simulink model "math_model_with_pid_2015a_the_newest"  (R2015a)
settings: Solver=ode3  SolverMode=SingleTasking  StartTime=0.0  StopTime=30  FixedStep=0.01  RelTol=1e-3
values from neighbouring files (symbols this model uses):
  f_c = 1.0942    [clean_pendulum_setup.m]
  f_p = 0.10436    [clean_pendulum_setup.m]
  g = 9.8101    [Wahadlo_setup.m]    (also in clean_pendulum_setup.m = 9.81)
  I = 1/12 * m_pw * l_c ^ 2      + 1/4 * m_pw * r_c ^ 2      + m_pw * l_c0 ^ 2      + 1/12 * m_ps * l_p ^ 2      + 1/4 * m_pw * r_p ^ 2      + m_ps * l_p0 ^ 2    (= 0.00542605689)    [clean_pendulum_setup.m]
  L = 0.2899    [clean_pendulum_setup.m]
  M = 0.503 + 0.045    (= 0.548)    [clean_pendulum_setup.m]
  m = m_c + m_p    (= 63.548)    [Wahadlo_setup.m]    (also in clean_pendulum_setup.m = 0.063)
  theta0 = pi/10    (= 0.314159265359)    [clean_pendulum_setup.m]
  theta_fin = 0    [clean_pendulum_setup.m]
  theta_max = pi    (= 3.14159265359)    [clean_pendulum_setup.m]
  x0 = -0.3    [clean_pendulum_setup.m]
  x_fin = 0    [clean_pendulum_setup.m]
  x_max = 0.75    [clean_pendulum_setup.m]
libraries: simulink x2
settings Model: CovMetricSettings=dwe  CovHtmlReporting=off  covSaveCumulativeToWorkspaceVar=off  CovSaveSingleToWorkspaceVar=off  CovExternalEMLEnable=on  Creator=spika  LastModifiedBy=Student
settings DataIOCC: LimitDataPoints=off  SaveFormat=Dataset  ReturnWorkspaceOutputs=on
settings DebuggingCC: SFUnexpectedBacktrackingDiag=error  SFNoUnconditionalDefaultTransitionDiag=error
settings HardwareCC: ProdBitPerPointer=64  ProdLargestAtomicFloat=Float  ProdIntDivRoundTo=Zero  ProdEndianess=LittleEndian  ProdHWDeviceType=Specified
settings ModelReferenceCC: PropagateSignalLabelsOutOfModel=on
settings SFSimCC: SimUseLocalCustomCode=on
settings RTWCC: RTWUseLocalCustomCode=on
settings GRTTargetCC: TargetLangStandard=C99 (ISO)

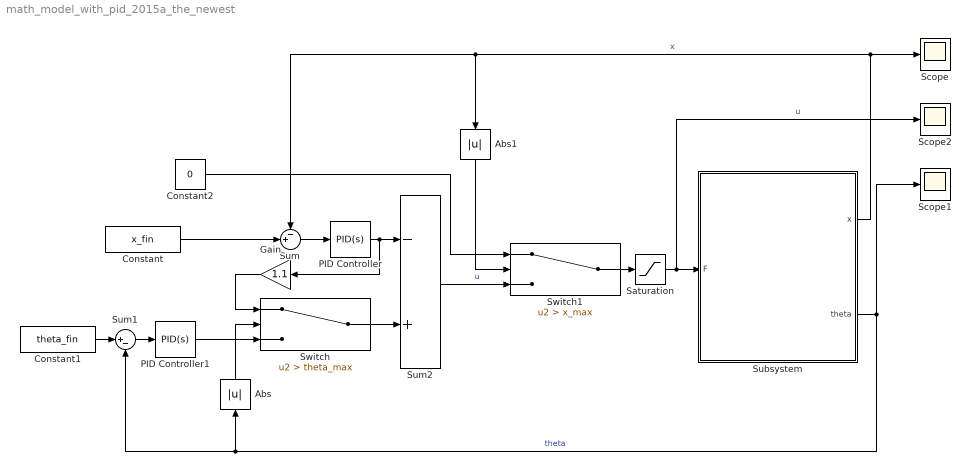
== system math_model_with_pid_2015a_the_newest ==
  Abs : Abs
  Abs1 : Abs
  Constant : Constant  Value=x_fin
  Constant1 : Constant  Value=theta_fin
  Constant2 : Constant  Value=0
  Gain : Gain  Gain=1.1
  PID Controller : simulink/Continuous/PID Controller  Controller=PID  TimeDomain=Continuous-time  SampleTime=-1  IntegratorMethod=Forward Euler  FilterMethod=Forward Euler  Form=Parallel  UseFilter=on  ControllerParametersSource=internal  P=0.9314  I=0  D=3.29  N=1.41571080218282  InitialConditionSource=internal  InitialConditionForIntegrator=0  InitialConditionForFilter=0  ExternalReset=none  LimitOutput=off  UpperSaturationLimit=inf  LowerSaturationLimit=-inf  LinearizeAsGain=on  AntiWindupMode=none  Kb=1  TrackingMode=off  Kt=1  PParamMin=[]  PParamMax=[]  IParamMin=[]  IParamMax=[]  DParamMin=[]  DParamMax=[]  NParamMin=[]  NParamMax=[]  KbParamMin=[]  KbParamMax=[]  KtParamMin=[]  KtParamMax=[]  POutMin=[]  POutMax=[]  IOutMin=[]  IOutMax=[]  DOutMin=[]  DOutMax=[]  NOutMin=[]  NOutMax=[]  KbOutMin=[]  KbOutMax=[]  KtOutMin=[]  KtOutMax=[]  IntegratorOutMin=[]  IntegratorOutMax=[]  FilterOutMin=[]  FilterOutMax=[]  SumOutMin=[]  SumOutMax=[]  SumI1OutMin=[]  SumI1OutMax=[]  SumI2OutMin=[]  SumI2OutMax=[]  SumI3OutMin=[]  SumI3OutMax=[]  SumDOutMin=[]  SumDOutMax=[]  SaturationOutMin=[]  SaturationOutMax=[]  IntegratorContinuousStateAttributes=''  IntegratorStateMustResolveToSignalObject=off  IntegratorRTWStateStorageClass=Auto  FilterContinuousStateAttributes=''  FilterStateMustResolveToSignalObject=off  FilterRTWStateStorageClass=Auto  DifferentiatorICPrevScaledInput=0  DifferentiatorOutMin=[]  DifferentiatorOutMax=[]
  PID Controller1 : simulink/Continuous/PID Controller  Controller=PID  TimeDomain=Continuous-time  SampleTime=-1  IntegratorMethod=Forward Euler  FilterMethod=Forward Euler  Form=Parallel  UseFilter=on  ControllerParametersSource=internal  P=-35  I=0  D=10  N=0.2  InitialConditionSource=internal  InitialConditionForIntegrator=0  InitialConditionForFilter=0  ExternalReset=none  LimitOutput=off  UpperSaturationLimit=inf  LowerSaturationLimit=-inf  LinearizeAsGain=on  AntiWindupMode=none  Kb=1  TrackingMode=off  Kt=1  PParamMin=[]  PParamMax=[]  IParamMin=[]  IParamMax=[]  DParamMin=[]  DParamMax=[]  NParamMin=[]  NParamMax=[]  KbParamMin=[]  KbParamMax=[]  KtParamMin=[]  KtParamMax=[]  POutMin=[]  POutMax=[]  IOutMin=[]  IOutMax=[]  DOutMin=[]  DOutMax=[]  NOutMin=[]  NOutMax=[]  KbOutMin=[]  KbOutMax=[]  KtOutMin=[]  KtOutMax=[]  IntegratorOutMin=[]  IntegratorOutMax=[]  FilterOutMin=[]  FilterOutMax=[]  SumOutMin=[]  SumOutMax=[]  SumI1OutMin=[]  SumI1OutMax=[]  SumI2OutMin=[]  SumI2OutMax=[]  SumI3OutMin=[]  SumI3OutMax=[]  SumDOutMin=[]  SumDOutMax=[]  SaturationOutMin=[]  SaturationOutMax=[]  IntegratorContinuousStateAttributes=''  IntegratorStateMustResolveToSignalObject=off  IntegratorRTWStateStorageClass=Auto  FilterContinuousStateAttributes=''  FilterStateMustResolveToSignalObject=off  FilterRTWStateStorageClass=Auto  DifferentiatorICPrevScaledInput=0  DifferentiatorOutMin=[]  DifferentiatorOutMax=[]
  Saturation : Saturate  UpperLimit=5  LowerLimit=-5
  Scope : Scope
      settings: YMin=-0.91693  YMax=0.61543
  Scope1 : Scope
      settings: YMin=-3.76605  YMax=-2.49503  SaveName=ScopeData2
  Scope2 : Scope
      settings: YMin=-6.25  YMax=6.25
  Subsystem : Subsystem
  Sum : Sum  Inputs=-+|
  Sum1 : Sum  Inputs=|+-
  Sum2 : Sum  Inputs=-+
  Switch : Switch  Criteria=u2 > Threshold  Threshold=theta_max
  Switch1 : Switch  Criteria=u2 > Threshold  Threshold=x_max
  wires:
  Subsystem/1(x) -> Sum/1, Abs1/1, Scope/1  "x"
  Subsystem/2(theta) -> Sum1/2, Abs/1, Scope1/1  "theta"
  Constant1/1 -> Sum1/1
  Constant/1 -> Sum/2
  Sum/1 -> PID Controller/1
  Sum1/1 -> PID Controller1/1
  PID Controller1/1 -> Switch/3
  Constant2/1 -> Switch1/1
  PID Controller/1 -> Gain/1, Sum2/1
  Abs/1 -> Switch/2
  Saturation/1 -> Subsystem/1(F), Scope2/1  "u"
  Switch/1 -> Sum2/2
  Switch1/1 -> Saturation/1
  Abs1/1 -> Switch1/2
  Sum2/1 -> Switch1/3  "u"
  Gain/1 -> Switch/1

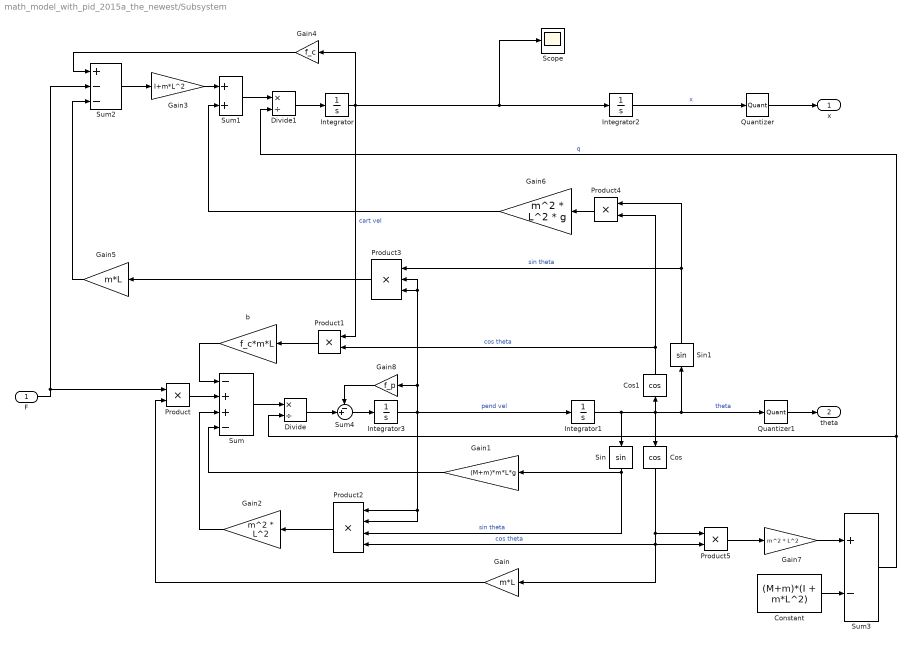
== system math_model_with_pid_2015a_the_newest/Subsystem ==
  F : Inport
  Constant : Constant  Value=(M+m)*(I + m*L^2)
  Cos : Trigonometry  Operator=cos
  Cos1 : Trigonometry  Operator=cos
  Divide : Product  Inputs=*/
  Divide1 : Product  Inputs=*/
  Gain : Gain  Gain=m*L
  Gain1 : Gain  Gain=(M+m)*m*L*g
  Gain2 : Gain  Gain=m^2 * L^2
  Gain3 : Gain  Gain=I+m*L^2
  Gain4 : Gain  Gain=f_c
  Gain5 : Gain  Gain=m*L
  Gain6 : Gain  Gain=m^2 * L^2 * g
  Gain7 : Gain  Gain=m^2 * L^2
  Gain8 : Gain  Gain=f_p
  Integrator : Integrator
  Integrator1 : Integrator  InitialCondition=theta0
  Integrator2 : Integrator  InitialCondition=x0
  Integrator3 : Integrator
  Product{,1,4..5} (4 alike) : Product
  Product2 : Product  Inputs=4
  Product3 : Product  Inputs=3
  Quantizer : Quantizer  QuantizationInterval=0.002
  Quantizer1 : Quantizer  QuantizationInterval=0.006
  Scope : Scope
      settings: YMin=-1.00000  YMax=1.00000  SaveName=ScopeData2
  Sin : Trigonometry
  Sin1 : Trigonometry
  Sum : Sum  Inputs=-++-
  Sum1 : Sum
  Sum2 : Sum  Inputs=+--
  Sum3 : Sum  Inputs=+-
  Sum4 : Sum  Inputs=-+|
  b : Gain  Gain=f_c*m*L
  x : Outport
  theta : Outport  Port=2
  wires:
  Integrator3/1 -> Product3/2, Product3/3, Gain8/1, Integrator1/1, Product2/1, Product2/2  "pend vel"
  Gain6/1 -> Sum1/2
  Gain3/1 -> Sum1/1
  Product1/1 -> b/1
  Integrator1/1 -> Cos1/1, Quantizer1/1, Sin1/1, Cos/1, Sin/1  "theta"
  Gain2/1 -> Sum/3
  Sin/1 -> Product2/3, Gain1/1  "sin theta"
  Product4/1 -> Gain6/1
  Sum2/1 -> Gain3/1
  Cos/1 -> Product5/1, Product5/2, Product2/4, Gain/1  "cos theta"
  b/1 -> Sum/1
  Sum/1 -> Divide/1
  Product/1 -> Sum/2
  Sum3/1 -> Divide1/2, Divide/2  "q"
  Integrator/1 -> Gain4/1, Scope/1, Integrator2/1, Product1/1  "cart vel"
  Sin1/1 -> Product4/1, Product3/1  "sin theta"
  Cos1/1 -> Product4/2, Product1/2  "cos theta"
  Sum1/1 -> Divide1/1
  Gain7/1 -> Sum3/1
  Gain1/1 -> Sum/4
  Gain8/1 -> Sum4/1
  Divide/1 -> Sum4/2
  Gain4/1 -> Sum2/1
  Product5/1 -> Gain7/1
  Sum4/1 -> Integrator3/1
  F/1 -> Sum2/2, Product/1
  Gain5/1 -> Sum2/3
  Gain/1 -> Product/2
  Constant/1 -> Sum3/2
  Product3/1 -> Gain5/1
  Integrator2/1 -> Quantizer/1  "x"
  Product2/1 -> Gain2/1
  Divide1/1 -> Integrator/1
  Quantizer/1 -> x/1
  Quantizer1/1 -> theta/1
